simulink model "ppm_psk_shared_v3"  (R2025a)
settings: Solver=VariableStepAuto  StartTime=0.0  StopTime=5e-6  RelTol=1e-3
model workspace (MAT data in the model file):
  Sig = Simulink.Signal
  Sig.Dimensions = -1
  Sig.DimensionsMode = 'auto'
  Sig.Complexity = 'auto'
  Sig.SampleTime = -1
  Sig.SamplingMode = 'auto'
  Sig.DataType = 'auto'
  Var = 0
  fc = 4000000000
  fs = 32000000000
  fsymbol = 500000000
  ppm_spacings2_ps = [-51.8 33.2 115.3 201.3 293.8 377.9 462.9 544.9]
  ppm_spacings_ps = [698 782 869 950 1045 1127 1210 1299]
  up_fs = 1024000000000
undefined symbols (not defined in the file or in its folder): PSK
libraries: dspsigops x11, simulink_extras x7, dspstat3 x5, commsink2 x3, dspfdesign x3, commchan3 x2, commrfcorlib x1, commdigbbndpm3 x1
settings Model: ParameterArgumentNames=ppm_spacings2_ps,ppm_spacings_ps  Creator=IWMAI  LastModifiedBy=IWMAI

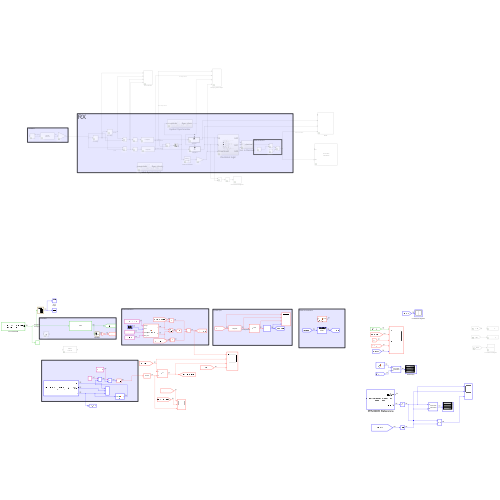
[thumbnail: Simulink's stored preview of the top-level diagram]
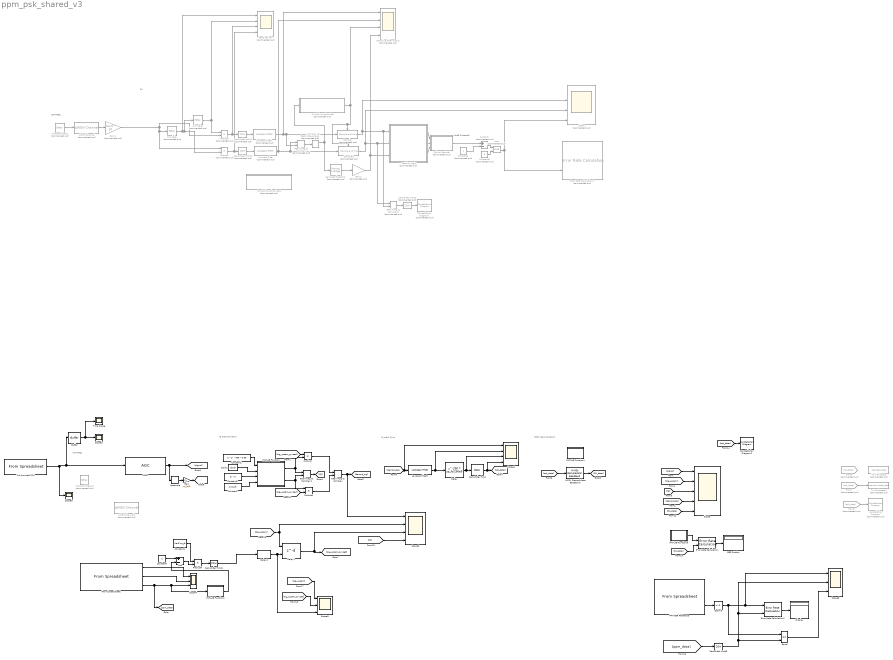
== system ppm_psk_shared_v3 ==
  note: Symbol Sync
  note: IQ Demodulation
  note: 8PSK Demodulation
  note: CHANNEL
  note: Mod8 Subtract1
  note: RX
  note: CHANNEL
  1ns trimmed PPM : FromSpreadsheet  FileName=C:\Users\IWMAI\University of Toronto\Yu Huang - Summer-2025-sharted\Yongkang\v5_250626\csv\phase_noise_ppm32.csv  SheetName=phase_noise_ppm32  SampleTime=1/fs  InterpolationWithinTimeRange=Zero order hold
  2ns delay : TransportDelay  Commented=on  DelayTime=1/fsymbol  FixedBuffer=on
  3bit to Decimal : Subsystem  Commented=on
  AGC1 : commrfcorlib/AGC  LegacyMode=off  DetectorMethod=Rectifier  LoopMethod=Linear  UpdatePeriod=100  StepSize=0.1  AdaptationStepSize=0.01  DesiredOutputPower=1  AveragingLength=100  MaximumGain=30  MaxPowerGain=60  GainOutputPort=off  InputPowerOutputPort=off  SimulateUsing=Interpreted execution
  AWGN Channel : commchan3/AWGN Channel  Commented=on  LegacyMode=off  NoiseMethod="Signal to noise ratio  (SNR)"  noiseMode="Signal to noise ratio  (SNR)"  EbNo=10  EsNo=10  SNR=16  BitsPerSymbol=1  SignalPower=1  SpecifySymbolPeriod=off  SamplesPerSymbol=1  SymbolPeriod=1  VarianceSource=Parameter  Variance=1  RandomStream=Global stream  Seed=67  SimulateUsing=Code generation
  AWGN Channel1 : commchan3/AWGN Channel  Commented=on  LegacyMode=off  NoiseMethod="Signal to noise ratio  (SNR)"  noiseMode="Signal to noise ratio  (SNR)"  EbNo=10  EsNo=10  SNR=16  BitsPerSymbol=1  SignalPower=3e-3  SpecifySymbolPeriod=off  SamplesPerSymbol=1  SymbolPeriod=1  VarianceSource=Parameter  Variance=1  RandomStream=Global stream  Seed=67  SimulateUsing=Code generation
  Add : Sum  Inputs=+-
  BER Display : Display
  Buffer : Buffer  N=32  OutputFrames=off
  Calibrate threshold : dspstat3/Moving Average  Commented=on  Method=Sliding window  ForgettingFactorPort=off  SpecifyWindowLength=on  WindowLength=10*fs/fsymbol  OverlapLength=10*fs/fsymbol - 1  AllowArbitraryInputLength=off  ForgettingFactor=0.9  SimulateUsing=Interpreted execution
  Clock1 : simulink_extras/Flip Flops/Clock  period=1/500e6
  Complex to Magnitude-Angle1 : ComplexToMagnitudeAngle  Commented=on
  Constant : Constant  Value=1/up_fs
  Constant1 : Constant  Value=2 * pi * 4e9 * 0.99
  Constant2 : Constant  Value=pi * 0
  Constant4 : Constant  Value=1e-9*up_fs
  Constant5 : Constant  Commented=on  Value=8
  Constant6 : Constant  Commented=on
  Constant7 : Constant  Value=2
  Constellation Diagram : ConstellationDiagram  Commented=on  WindowPosition=[70.000000,304.000000,385.000000,254.000000,]  ScopeFrameLocation=window  SymbolsToDisplaySource=Property  SymbolsToDisplay=2500  ReferenceConstellation=8-PSK  XLimits=[-2.067197093509777,2.1540515483355467]  YLimits=[-2.067197093509777,2.1540515483355467]  AxesLimits=[-2.067197093509777,2.1540515483355467]  EnableMeasurements=on  DefaultConfigurationName=comm.scopes.ConstellationDiagramBlockCfg
  Constellation Diagram1 : ConstellationDiagram  Commented=on  WindowPosition=[363.000000,63.000000,600.000000,600.000000,]  ScopeFrameLocation=window  SymbolsToDisplaySource=Property  SymbolsToDisplay=1000  XLimits=[-1.58,1.61]  YLimits=[-1.58,1.61]  AxesLimits=[-1.58,1.61]  EnableMeasurements=on
  Constellation Diagram2 : ConstellationDiagram  WindowPosition=[198.000000,182.000000,773.000000,552.000000,]  ScopeFrameLocation=window  SymbolsToDisplaySource=Property  SymbolsToDisplay=2500  ShowLegend=on  MaximizeAxes=on  DefaultConfigurationName=comm.scopes.ConstellationDiagramBlockCfg
  Datas : Scope  Commented=on  NumInputPorts=4
      settings: ActiveDisplayYMinimum=-0.875  ActiveDisplayYMaximum=7.875  DataLoggingVariableName=ScopeData4
  Decision logic : Subsystem  Commented=on
  Delay : Delay  DelayLength=290 * up_fs/256e9  DelayLengthUpperLimit=512  InputProcessing=Columns as channels (frame based)
  Delay1 : Delay  DelayLengthSource=Input port  DelayLength=1  DelayLengthUpperLimit=2*up_fs/1e9  InputProcessing=Columns as channels (frame based)
      settings: InputPortMap=u0,p1
  Delay2 : Delay  DelayLength=1e-9*up_fs
  Delay3 : Delay  DelayLength=0
  Display : Display
  Equal : RelationalOperator  Operator===  OutDataTypeStr=boolean  RndMeth=Simplest  InputSameDT=off
  Error Rate Calculation : commsink2/Error Rate Calculation  N=0  st_delay=0  cp_mode=Entire frame  subframe=[]  PMode=Port  WsName=ErrorVec  RsMode2=off  stop=off  numErr=100  maxBits=1e6
      settings: LibrarySourceBlock=|
      | commhdlsink/Error Rate
      | Calculation
  Error Rate Calculation1 : commsink2/Error Rate Calculation  Commented=on  N=1  st_delay=0  cp_mode=Entire frame  subframe=[]  PMode=Workspace  WsName=ErrorVec  RsMode2=off  stop=off  numErr=100  maxBits=1e6
  Error Rate Calculation2 : commsink2/Error Rate Calculation  N=0  st_delay=0  cp_mode=Entire frame  subframe=[]  PMode=Port  WsName=ErrorVec  RsMode2=off  stop=off  numErr=100  maxBits=1e6
      settings: LibrarySourceBlock=|
      | commhdlsink/Error Rate
      | Calculation
  From Spreadsheet : FromSpreadsheet  FileName=C:\Users\IWMAI\University of Toronto\Yu Huang - Summer-2025-sharted\Yongkang\v5_250626\csv\ppm_decode.csv  SheetName=ppm_decode  TreatFirstColumnAs=Data  SampleTime=1/fsymbol
  From7 : From  Commented=on  GotoTag=psk_data
  From8 : From  Commented=on  GotoTag=psk_data
  From9 : From  Commented=on  GotoTag=RX_data
  Gain : Gain  Gain=up_fs/fs
  Gain1 : Gain  Commented=on  Gain=rand * 10
  Gain2 : Gain  Commented=on  Gain=1/sqrt(2)
  Lowpass Filter : dspfdesign/Lowpass Filter  Commented=on  FilterType=FIR  DesignForMinimumOrder=on  FilterOrder=50  PassbandFrequency=0.05*fc  StopbandFrequency=0.6*fc  PassbandRipple=0.1  StopbandAttenuation=80  SampleRateMode=Specify on dialog  SampleRate=fs  SimulateUsing=Interpreted execution  roundingMode=Floor  coeffsDataTypeStr=fixdt(1,16)
  Lowpass Filter1 : dspfdesign/Lowpass Filter  Commented=on  FilterType=FIR  DesignForMinimumOrder=on  FilterOrder=50  PassbandFrequency=0.05*fc  StopbandFrequency=0.6*fc  PassbandRipple=0.1  StopbandAttenuation=80  SampleRateMode=Specify on dialog  SampleRate=fs  SimulateUsing=Interpreted execution  roundingMode=Floor  coeffsDataTypeStr=fixdt(1,16)
  Lowpass Filter3 : dspfdesign/Lowpass Filter  FilterType=FIR  DesignForMinimumOrder=on  FilterOrder=50  PassbandFrequency=0.05*fc  StopbandFrequency=0.6*fc  PassbandRipple=0.1  StopbandAttenuation=80  SampleRate=fs  SimulateUsing=Interpreted execution  roundingMode=Floor  coeffsDataTypeStr=fixdt(1,16)
  M-PSK Demodulator Baseband : commdigbbndpm3/M-PSK Demodulator Baseband  M=8  OutType=Integer  DecType=Hard decision  VarSource=Dialog  Variance=1  Dec=Gray  Mapping=[0:7]  Ph=pi/8  outDtype1=Inherit via internal rule  outDtype2=Inherit via internal rule  derotateFactorWordLen=16  derotateFactorDataTypeStr=Inherit: Same word length as input  derotateFactorLastDataTypeStr=Inherit: Same word length as input
      settings: LibrarySourceBlock=|
      | commhdldigbbndpm/M-PSK
      | Demodulator
      | Baseband
  MATLAB Function : MATLAB Function  TreatAsAtomicUnit=on  SystemSampleTime=1/up_fs
  MATLAB Function1 : MATLAB Function  TreatAsAtomicUnit=on
  MATLAB Function3 : MATLAB Function  TreatAsAtomicUnit=on  SystemSampleTime=1/500e6
  MATLAB Function4 : MATLAB Function  TreatAsAtomicUnit=on
  Mod : Math  Commented=on  Operator=mod
  PPM BER Reference : FromSpreadsheet  FileName=C:\Users\IWMAI\University of Toronto\Yu Huang - Summer-2025-sharted\Yongkang\v5_250626\csv\ground_truth_ppm.csv  SheetName=ground_truth_ppm  TreatFirstColumnAs=Data  SampleTime=1/fsymbol
  Product : Product
  Product1 : Product
  Product2 : Product  Commented=on
  Product3 : Product  Commented=on
  Product4 : Product
  Real-Imag to Complex : RealImagToComplex
  Real-Imag to Complex1 : RealImagToComplex
  Real-Imag to Complex2 : RealImagToComplex  Commented=on
  Real-Imag to Complex3 : RealImagToComplex  Commented=on
  Received raw : Scope  Commented=on  NumInputPorts=4
      settings: ActiveDisplayYMinimum=-8.64062  ActiveDisplayYMaximum=9.0483  DataLoggingVariableName=ScopeData5
  Sampler : dspsigops/Sample and Hold  Commented=on  trig=Rising edge  initCond=0  latchinput=off
  Sampler1 : dspsigops/Sample and Hold  Commented=on  trig=Rising edge  initCond=0  latchinput=off
  Sampling Filter output : Scope  Commented=on  NumInputPorts=4
      settings: ActiveDisplayYMinimum=-6.30438  ActiveDisplayYMaximum=6.9861  DataLoggingVariableName=ScopeData6
  Scope : Scope  NumInputPorts=5
      settings: ActiveDisplayYMinimum=-3.2971710288295304  ActiveDisplayYMaximum=3.6439303524490732
  Scope1 : Scope  NumInputPorts=4
      settings: ActiveDisplayYMinimum=-217.12328360095091  ActiveDisplayYMaximum=190.25679951109339  DataLoggingVariableName=ScopeData3
  Scope2 : Scope
      settings: ActiveDisplayYMinimum=-1  ActiveDisplayYMaximum=1  DataLoggingVariableName=ScopeData7
  Scope3 : Scope  NumInputPorts=4
      settings: ActiveDisplayYMinimum=-121.24929806481079  ActiveDisplayYMaximum=113.85916593857471  DataLoggingVariableName=ScopeData11
  Scope4 : Scope  NumInputPorts=3
      settings: ActiveDisplayYMinimum=-62.374999999999986  ActiveDisplayYMaximum=561.375  DataLoggingVariableName=ScopeData13
  Scope5 : Scope
      settings: ActiveDisplayYMinimum=-3.5739980150661266  ActiveDisplayYMaximum=0.60767584738395508  DataLoggingVariableName=ScopeData14
  Scope8 : Scope  NumInputPorts=3
      settings: ActiveDisplayYMinimum=-0.87499999999999978  ActiveDisplayYMaximum=7.875  DataLoggingVariableName=ScopeData17
  Scope9 : Scope  NumInputPorts=3
      settings: ActiveDisplayYMinimum=-2041.2616026203843  ActiveDisplayYMaximum=448.10816733090951  DataLoggingVariableName=ScopeData18
  Subtract : Sum  Commented=on  Inputs=+-
  Symbol Synchronizer : Subsystem  Commented=on
  Symbol Synchronizer1 : Subsystem  Commented=on
  Time Scope : Scope
      settings: TimeUnits=Metric (based on Time Span)  ActiveDisplayYMinimum=-0.20228703271248236  ActiveDisplayYMaximum=0.23303505029941141  YLabel=Amplitude  DataLoggingVariableName=ScopeData8
  To Workspace : ToWorkspace  Commented=on  VariableName=decoded_data  SaveFormat=Structure With Time  SampleTime=-1
  To Workspace1 : ToWorkspace  Commented=on  VariableName=demodulated_data  SaveFormat=Structure With Time  SampleTime=-1
  Transport Delay : TransportDelay  Commented=on  DelayTime=rand * pi/fsymbol
  Transport Delay3 : TransportDelay  Commented=on  DelayTime=rand * pi/fsymbol
  Upsample : dspsigops/Upsample  FactorSource=Dialog parameter  N=up_fs/fs  Nmax=16  phase=0  RateOptions=Allow multirate processing  ic=0  mode=Unused parameter value
      settings: LibrarySourceBlock=dsphdlsupportsigops/Upsample
  Zero-Order Hold : ZeroOrderHold  SampleTime=1/fsymbol
  Zero-Order Hold1 : ZeroOrderHold  Commented=on  SampleTime=1/fsymbol
  Zero-Order Hold2 : ZeroOrderHold  Commented=on  SampleTime=1/fs
  Zero-Order Hold3 : ZeroOrderHold  Commented=on  SampleTime=1/fs
  Zero-Order Hold4 : ZeroOrderHold  SampleTime=1/up_fs
  Zero-Order Hold5 : ZeroOrderHold  SampleTime=1/fsymbol
  pi/2 delay : TransportDelay  Commented=on  DelayTime=1/(fc)/4  FixedBuffer=on
  wires:
  From8/1 -> Constellation Diagram/1
  MATLAB Function3/1(y) -> Error Rate Calculation/1
  Error Rate Calculation/1 -> BER Display/1
  2ns delay/1 -> Product2/2, pi/2 delay/1, Received raw/1  "I p ath"
  Symbol Synchronizer/1(Sync. clock) -> Sampling Filter output/3, Sampler/Trigger, Sampler1/Trigger
  Sampler/1 -> Real-Imag to Complex3/2, Decision logic/1(Q), Datas/2
  Mod/1 -> Error Rate Calculation1/2, Datas/4  "Recovered data"
  pi/2 delay/1 -> Received raw/2, Product3/1  "Q path"
  3bit to Decimal/1(decimal) -> Subtract/1
  Decision logic/2(bit1) -> 3bit to Decimal/2(In2)
  Sampler1/1 -> Datas/3, Real-Imag to Complex3/1, Decision logic/2(I)
  Product3/1 -> Zero-Order Hold2/1, Received raw/3
  Decision logic/3(bit2) -> 3bit to Decimal/3(In3)
  Complex to Magnitude-Angle1/1 -> Symbol Synchronizer/1(magnitude), Calibrate threshold/1
  AWGN Channel/1 -> Gain1/1  "RX"
  Zero-Order Hold3/1 -> Lowpass Filter/1
  Transport Delay/1 -> AWGN Channel/1  "RX Signal"
  Subtract/1 -> Mod/1
  Real-Imag to Complex2/1 -> Complex to Magnitude-Angle1/1
  Lowpass Filter/1 -> Real-Imag to Complex2/1, Sampler1/1, Sampling Filter output/2  "no delay filtered"
  Constant5/1 -> Mod/2
  Gain2/1 -> Sampling Filter output/4, Decision logic/3(threshhold)
  Calibrate threshold/1 -> Gain2/1
  Product2/1 -> Zero-Order Hold3/1, Received raw/4
  Gain1/1 -> Product2/1, 2ns delay/1, Product3/2
  Constant6/1 -> Subtract/2
  Decision logic/1(bit0) -> 3bit to Decimal/1(In1)
  Zero-Order Hold1/1 -> Constellation Diagram1/1
  Real-Imag to Complex3/1 -> Zero-Order Hold1/1
  Zero-Order Hold2/1 -> Lowpass Filter1/1
  Lowpass Filter1/1 -> Sampling Filter output/1, Real-Imag to Complex2/2, Sampler/1  "90o delay filtered"
  [signal] -> Scope/1
  [IQ] -> Scope/3
  [demod_sig] -> Scope1/1, Lowpass Filter3/1
  Zero-Order Hold/1 -> Scope1/4, [psk_data]
  [psk_data] -> M-PSK Demodulator Baseband/1
  From7/1 -> To Workspace1/1
  M-PSK Demodulator Baseband/1 -> [RX_data]
  [RX_data] -> Error Rate Calculation/2
  Real-Imag to Complex1/1 -> [IQ]
  Constant1/1 -> MATLAB Function/1(omega)
  Clock1/1 -> MATLAB Function/2(clock)
  Constant2/1 -> MATLAB Function/3(phase_shift)
  MATLAB Function/1(I) -> Real-Imag to Complex1/1, Product/2
  MATLAB Function/2(Q) -> Product1/1, Real-Imag to Complex1/2
  [sig_upsam_synced] -> Product/1
  [sig_upsam_synced] -> Product1/2
  Product/1 -> Real-Imag to Complex/1
  Product1/1 -> Real-Imag to Complex/2
  Real-Imag to Complex/1 -> Scope3/1, [demod_sig]
  [demod_sig] -> Scope/4
  [RX_data] -> Scope/5
  1ns trimmed PPM/1 -> AGC1/1, Buffer/1, Scope5/1  "RX Signal"
  AGC1/1 -> Upsample/1, [signal]
  Buffer/1 -> Time Scope/1, Scope2/1
  Constant/1 -> MATLAB Function/4(delta_time)
  Lowpass Filter3/1 -> Scope1/2, Delay/1  "no delay filtered"
  Upsample/1 -> Gain/1
  [sig_upsam] -> Scope/2
  From Spreadsheet/1 -> Scope4/1
  From Spreadsheet/2 -> Scope4/2
  From Spreadsheet/3 -> [ppm_data], MATLAB Function1/1(index), Scope4/3
  Constant4/1 -> Product4/1
  Constant7/1 -> Add/1
  Add/1 -> Product4/2
  Delay/1 -> Scope1/3, Zero-Order Hold/1
  Product4/1 -> Zero-Order Hold4/1
  [sig_upsam] -> Delay1/1, Scope3/2
  Delay1/1 -> [sig_upsam_synced], Scope3/3
  Zero-Order Hold4/1 -> Delay2/1
  Delay2/1 -> Scope9/3, Delay1/2
  [psk_data] -> Constellation Diagram2/1
  Gain/1 -> [sig_upsam]
  [IQ] -> Scope3/4
  PPM BER Reference/2 -> Delay3/1
  Equal/1 -> Scope8/3
  Error Rate Calculation2/1 -> Display/1
  Zero-Order Hold5/1 -> Scope8/2, Error Rate Calculation2/2, Equal/2
  Delay3/1 -> Scope8/1, Error Rate Calculation2/1, Equal/1
  [ppm_data] -> Zero-Order Hold5/1
  [sig_upsam] -> Scope9/1
  [sig_upsam_synced] -> Scope9/2
  MATLAB Function1/1(y) -> Add/2

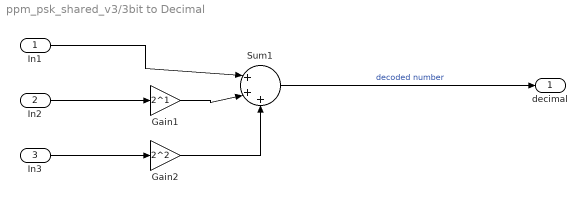
== system ppm_psk_shared_v3/3bit to Decimal ==
  In1 : Inport
  In2 : Inport  Port=2
  In3 : Inport  Port=3
  Gain1 : Gain  Gain=2^1
  Gain2 : Gain  Gain=2^2
  Sum1 : Sum  Inputs=|+++
  decimal : Outport
  wires:
  Gain2/1 -> Sum1/3
  Gain1/1 -> Sum1/2
  In3/1 -> Gain2/1
  In1/1 -> Sum1/1
  In2/1 -> Gain1/1
  Sum1/1 -> decimal/1  "decoded number"

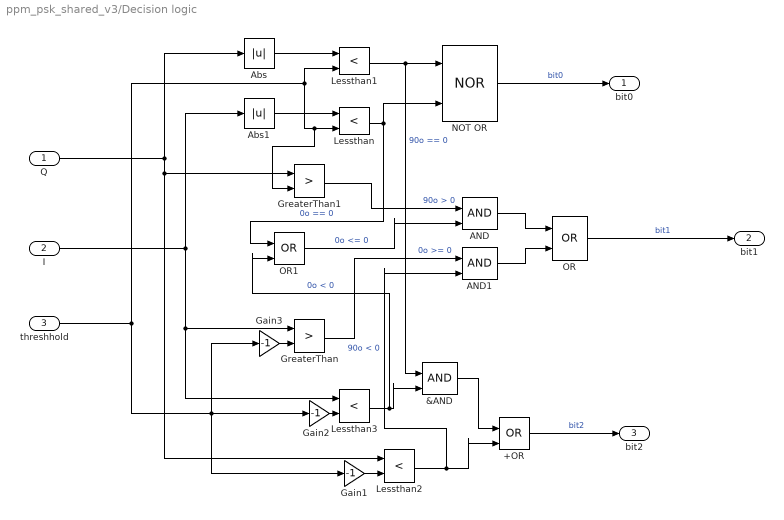
== system ppm_psk_shared_v3/Decision logic ==
  Q : Inport
  I : Inport  Port=2
  threshhold : Inport  Port=3
  &AND : Logic  IconShape=distinctive  AllPortsSameDT=off  OutDataTypeStr=boolean
  +OR : Logic  Operator=OR  IconShape=distinctive  AllPortsSameDT=off  OutDataTypeStr=boolean
  AND : Logic  IconShape=distinctive  AllPortsSameDT=off  OutDataTypeStr=boolean
  AND1 : Logic  IconShape=distinctive  AllPortsSameDT=off  OutDataTypeStr=boolean
  Abs : Abs  SaturateOnIntegerOverflow=off
  Abs1 : Abs  SaturateOnIntegerOverflow=off
  Gain1 : Gain  Gain=-1
  Gain2 : Gain  Gain=-1
  Gain3 : Gain  Gain=-1
  GreaterThan : RelationalOperator  Operator=>  OutDataTypeStr=boolean  RndMeth=Simplest  InputSameDT=off
  GreaterThan1 : RelationalOperator  Operator=>  OutDataTypeStr=boolean  RndMeth=Simplest  InputSameDT=off
  "Lessthan " : RelationalOperator  Operator=<  OutDataTypeStr=boolean  RndMeth=Simplest  InputSameDT=off
  Lessthan1 : RelationalOperator  Operator=<  OutDataTypeStr=boolean  RndMeth=Simplest  InputSameDT=off
  Lessthan2 : RelationalOperator  Operator=<  OutDataTypeStr=boolean  RndMeth=Simplest  InputSameDT=off
  Lessthan3 : RelationalOperator  Operator=<  OutDataTypeStr=boolean  RndMeth=Simplest  InputSameDT=off
  NOT OR : Logic  Operator=NOR  IconShape=distinctive  AllPortsSameDT=off  OutDataTypeStr=boolean
  OR : Logic  Operator=OR  IconShape=distinctive  AllPortsSameDT=off  OutDataTypeStr=boolean
  OR1 : Logic  Operator=OR  IconShape=distinctive  AllPortsSameDT=off  OutDataTypeStr=boolean
  bit0 : Outport
  bit1 : Outport  Port=2
  bit2 : Outport  Port=3
  wires:
  NOT OR/1 -> bit0/1  "bit0"
  Lessthan2/1 -> AND1/2, +OR/2  "90o < 0"
  "Lessthan "/1 -> OR1/1, NOT OR/2  "0o == 0"
  Abs1/1 -> "Lessthan "/1
  GreaterThan/1 -> AND1/1  "0o >= 0"
  I/1 -> Abs1/1, GreaterThan/1, Lessthan3/1
  Gain1/1 -> Lessthan2/2
  OR1/1 -> AND/2  "0o <= 0"
  GreaterThan1/1 -> AND/1  "90o > 0"
  AND/1 -> OR/1
  Q/1 -> Abs/1, Lessthan2/1, GreaterThan1/1
  Gain3/1 -> GreaterThan/2
  Lessthan3/1 -> OR1/2, &AND/2  "0o < 0"
  Abs/1 -> Lessthan1/1
  threshhold/1 -> Gain1/1, Gain2/1, Gain3/1, GreaterThan1/2, "Lessthan "/2, Lessthan1/2
  Lessthan1/1 -> NOT OR/1, &AND/1  "90o == 0"
  AND1/1 -> OR/2
  &AND/1 -> +OR/1
  Gain2/1 -> Lessthan3/2
  +OR/1 -> bit2/1  "bit2"
  OR/1 -> bit1/1  "bit1"

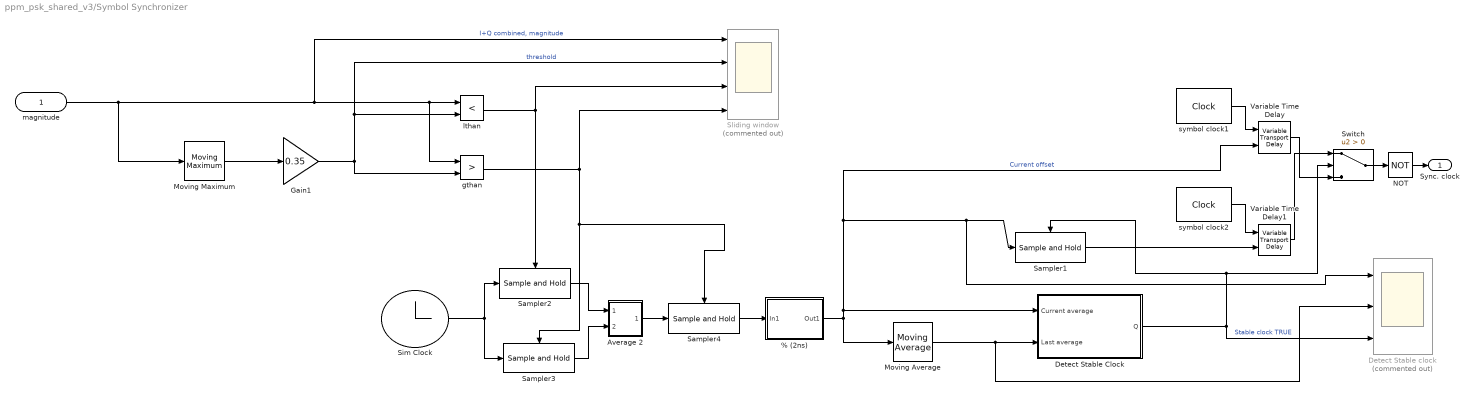
== system ppm_psk_shared_v3/Symbol Synchronizer ==
  magnitude : Inport
  % (2ns) : Subsystem
  Average 2 : Subsystem
  Detect Stable Clock : Subsystem
  Detect Stable clock : Scope  Commented=on  NumInputPorts=3
      settings: ActiveDisplayYMinimum=-1E-10  ActiveDisplayYMaximum=1.2E-9
  Gain1 : Gain  Gain=0.35
  Moving Average : dspstat3/Moving Average  Method=Sliding window  ForgettingFactorPort=off  SpecifyWindowLength=on  WindowLength=4*fs/fsymbol  OverlapLength=4*fs/fsymbol-1  AllowArbitraryInputLength=off  ForgettingFactor=0.9  SimulateUsing=Interpreted execution
  Moving Maximum : dspstat3/Moving Maximum  SpecifyWindowLength=on  WindowLength=2*fs/fsymbol  SimulateUsing=Interpreted execution
  NOT : Logic  Operator=NOT  IconShape=distinctive  AllPortsSameDT=off  OutDataTypeStr=boolean
  Sampler{1..4} (4 alike) : dspsigops/Sample and Hold  trig=Rising edge  initCond=0  latchinput=off
  Sim Clock : Clock
  Sliding window : Scope  Commented=on  NumInputPorts=4
      settings: ActiveDisplayYMinimum=-1.49431  ActiveDisplayYMaximum=13.44875  DataLoggingVariableName=ScopeData2
  Switch : Switch  Criteria=u2 > Threshold  SaturateOnIntegerOverflow=off  InputSameDT=off
  Variable Time Delay : VariableTransportDelay  MaximumDelay=10
  Variable Time Delay1 : VariableTransportDelay  MaximumDelay=10
  gthan : RelationalOperator  Operator=>  OutDataTypeStr=boolean  RndMeth=Simplest  InputSameDT=off
  lthan : RelationalOperator  Operator=<  OutDataTypeStr=boolean  RndMeth=Simplest  InputSameDT=off
  symbol clock1 : simulink_extras/Flip Flops/Clock  period=1/fsymbol
  symbol clock2 : simulink_extras/Flip Flops/Clock  period=1/fsymbol
  Sync. clock : Outport
  wires:
  Sim Clock/1 -> Sampler2/1, Sampler3/1
  Sampler3/1 -> Average 2/2(In2)
  Gain1/1 -> gthan/2, Sliding window/2, lthan/2  "threshold"
  Sampler2/1 -> Average 2/1(In1)
  symbol clock1/1 -> Variable Time Delay/1
  Sampler4/1 -> % (2ns)/1(In1)
  lthan/1 -> Sampler2/Trigger, Sliding window/3
  Average 2/1(Out1) -> Sampler4/1
  magnitude/1 -> Moving Maximum/1, Sliding window/1, gthan/1, lthan/1  "I+Q combined, magnitude"
  gthan/1 -> Sampler4/Trigger, Sampler3/Trigger, Sliding window/4
  symbol clock2/1 -> Variable Time Delay1/1
  Sampler1/1 -> Variable Time Delay1/2
  Switch/1 -> NOT/1
  Variable Time Delay/1 -> Switch/3
  Variable Time Delay1/1 -> Switch/1
  NOT/1 -> Sync. clock/1
  Detect Stable Clock/1(Q) -> Detect Stable clock/3, Sampler1/Trigger, Switch/2  "Stable clock TRUE"
  % (2ns)/1(Out1) -> Variable Time Delay/2, Detect Stable clock/1, Sampler1/1, Detect Stable Clock/1(Current average), Moving Average/1  "Current offset"
  Moving Maximum/1 -> Gain1/1
  Moving Average/1 -> Detect Stable clock/2, Detect Stable Clock/2(Last average)

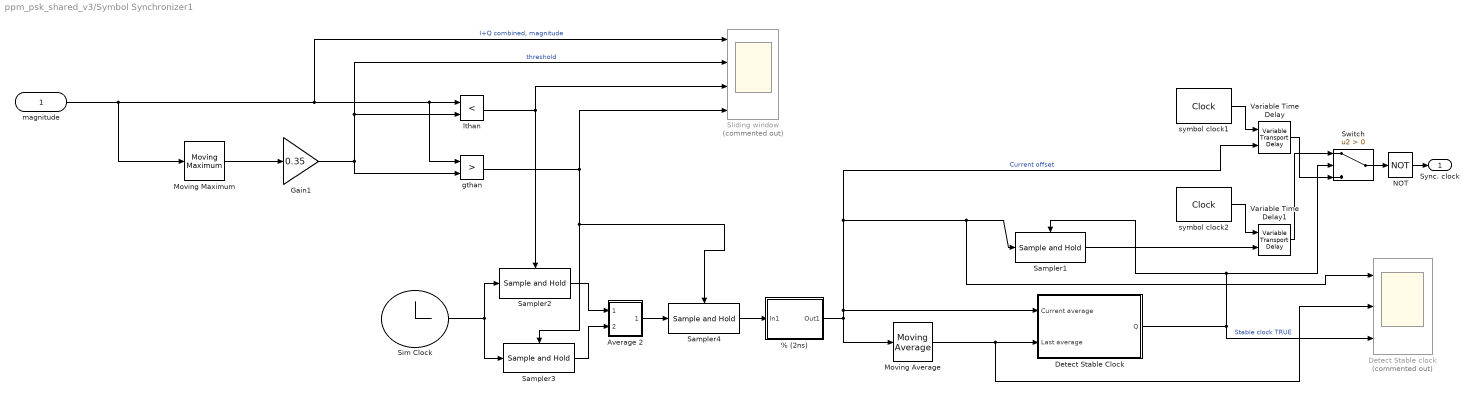
== system ppm_psk_shared_v3/Symbol Synchronizer1 ==
  magnitude : Inport
  % (2ns) : Subsystem
  Average 2 : Subsystem
  Detect Stable Clock : Subsystem
  Detect Stable clock : Scope  Commented=on  NumInputPorts=3
      settings: ActiveDisplayYMinimum=-1E-10  ActiveDisplayYMaximum=1.2E-9
  Gain1 : Gain  Gain=0.35
  Moving Average : dspstat3/Moving Average  Method=Sliding window  ForgettingFactorPort=off  SpecifyWindowLength=on  WindowLength=4*fs/fsymbol  OverlapLength=4*fs/fsymbol-1  AllowArbitraryInputLength=off  ForgettingFactor=0.9  SimulateUsing=Interpreted execution
  Moving Maximum : dspstat3/Moving Maximum  SpecifyWindowLength=on  WindowLength=2*fs/fsymbol  SimulateUsing=Interpreted execution
  NOT : Logic  Operator=NOT  IconShape=distinctive  AllPortsSameDT=off  OutDataTypeStr=boolean
  Sampler{1..4} (4 alike) : dspsigops/Sample and Hold  trig=Rising edge  initCond=0  latchinput=off
  Sim Clock : Clock
  Sliding window : Scope  Commented=on  NumInputPorts=4
      settings: ActiveDisplayYMinimum=-1.49431  ActiveDisplayYMaximum=13.44875  DataLoggingVariableName=ScopeData2
  Switch : Switch  Criteria=u2 > Threshold  SaturateOnIntegerOverflow=off  InputSameDT=off
  Variable Time Delay : VariableTransportDelay  MaximumDelay=10
  Variable Time Delay1 : VariableTransportDelay  MaximumDelay=10
  gthan : RelationalOperator  Operator=>  OutDataTypeStr=boolean  RndMeth=Simplest  InputSameDT=off
  lthan : RelationalOperator  Operator=<  OutDataTypeStr=boolean  RndMeth=Simplest  InputSameDT=off
  symbol clock1 : simulink_extras/Flip Flops/Clock  period=1/fsymbol
  symbol clock2 : simulink_extras/Flip Flops/Clock  period=1/fsymbol
  Sync. clock : Outport
  wires:
  Sim Clock/1 -> Sampler2/1, Sampler3/1
  Sampler3/1 -> Average 2/2(In2)
  Gain1/1 -> gthan/2, Sliding window/2, lthan/2  "threshold"
  Sampler2/1 -> Average 2/1(In1)
  symbol clock1/1 -> Variable Time Delay/1
  Sampler4/1 -> % (2ns)/1(In1)
  lthan/1 -> Sampler2/Trigger, Sliding window/3
  Average 2/1(Out1) -> Sampler4/1
  magnitude/1 -> Moving Maximum/1, Sliding window/1, gthan/1, lthan/1  "I+Q combined, magnitude"
  gthan/1 -> Sampler4/Trigger, Sampler3/Trigger, Sliding window/4
  symbol clock2/1 -> Variable Time Delay1/1
  Sampler1/1 -> Variable Time Delay1/2
  Switch/1 -> NOT/1
  Variable Time Delay/1 -> Switch/3
  Variable Time Delay1/1 -> Switch/1
  NOT/1 -> Sync. clock/1
  Detect Stable Clock/1(Q) -> Detect Stable clock/3, Sampler1/Trigger, Switch/2  "Stable clock TRUE"
  % (2ns)/1(Out1) -> Variable Time Delay/2, Detect Stable clock/1, Sampler1/1, Detect Stable Clock/1(Current average), Moving Average/1  "Current offset"
  Moving Maximum/1 -> Gain1/1
  Moving Average/1 -> Detect Stable clock/2, Detect Stable Clock/2(Last average)

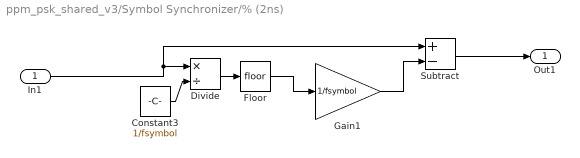
== system ppm_psk_shared_v3/Symbol Synchronizer/% (2ns) ==
  In1 : Inport
  Constant3 : Constant  Value=1/fsymbol
  Divide : Product  Inputs=*/
  Floor : Rounding
  Gain1 : Gain  Gain=1/fsymbol
  Subtract : Sum  Inputs=+-
  Out1 : Outport
  wires:
  Subtract/1 -> Out1/1
  Divide/1 -> Floor/1
  In1/1 -> Subtract/1, Divide/1
  Gain1/1 -> Subtract/2
  Floor/1 -> Gain1/1
  Constant3/1 -> Divide/2

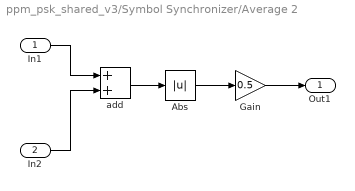
== system ppm_psk_shared_v3/Symbol Synchronizer/Average 2 ==
  In1 : Inport
  In2 : Inport  Port=2
  Abs : Abs  SaturateOnIntegerOverflow=off
  Gain : Gain  Gain=0.5
  add : Sum
  Out1 : Outport
  wires:
  Gain/1 -> Out1/1
  In1/1 -> add/1
  In2/1 -> add/2
  add/1 -> Abs/1
  Abs/1 -> Gain/1

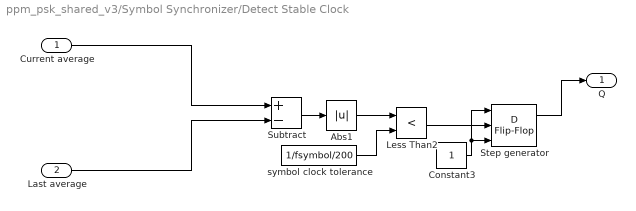
== system ppm_psk_shared_v3/Symbol Synchronizer/Detect Stable Clock ==
  Current average : Inport
  Last average : Inport  Port=2
  Abs1 : Abs  SaturateOnIntegerOverflow=off
  Constant3 : Constant  OutDataTypeStr=boolean
  Less Than2 : RelationalOperator  Operator=<  OutDataTypeStr=boolean  RndMeth=Simplest  InputSameDT=off
  Step generator : simulink_extras/Flip Flops/D Flip-Flop
  Subtract : Sum  Inputs=+-
  symbol clock tolerance : Constant  Value=1/fsymbol/200
  Q : Outport
  wires:
  symbol clock tolerance/1 -> Less Than2/2
  Subtract/1 -> Abs1/1
  Constant3/1 -> Step generator/1, Step generator/3
  Last average/1 -> Subtract/2
  Abs1/1 -> Less Than2/1
  Less Than2/1 -> Step generator/2
  Step generator/1 -> Q/1
  Current average/1 -> Subtract/1

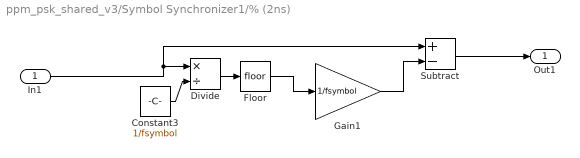
== system ppm_psk_shared_v3/Symbol Synchronizer1/% (2ns) ==
  In1 : Inport
  Constant3 : Constant  Value=1/fsymbol
  Divide : Product  Inputs=*/
  Floor : Rounding
  Gain1 : Gain  Gain=1/fsymbol
  Subtract : Sum  Inputs=+-
  Out1 : Outport
  wires:
  Subtract/1 -> Out1/1
  Divide/1 -> Floor/1
  In1/1 -> Subtract/1, Divide/1
  Gain1/1 -> Subtract/2
  Floor/1 -> Gain1/1
  Constant3/1 -> Divide/2

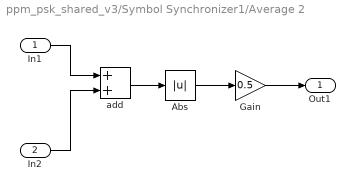
== system ppm_psk_shared_v3/Symbol Synchronizer1/Average 2 ==
  In1 : Inport
  In2 : Inport  Port=2
  Abs : Abs  SaturateOnIntegerOverflow=off
  Gain : Gain  Gain=0.5
  add : Sum
  Out1 : Outport
  wires:
  Gain/1 -> Out1/1
  In1/1 -> add/1
  In2/1 -> add/2
  add/1 -> Abs/1
  Abs/1 -> Gain/1

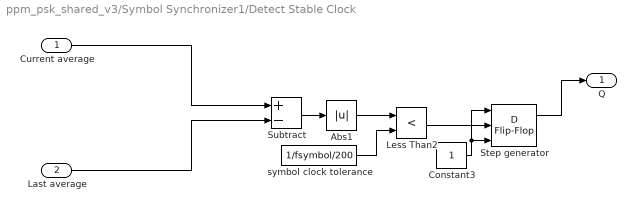
== system ppm_psk_shared_v3/Symbol Synchronizer1/Detect Stable Clock ==
  Current average : Inport
  Last average : Inport  Port=2
  Abs1 : Abs  SaturateOnIntegerOverflow=off
  Constant3 : Constant  OutDataTypeStr=boolean
  Less Than2 : RelationalOperator  Operator=<  OutDataTypeStr=boolean  RndMeth=Simplest  InputSameDT=off
  Step generator : simulink_extras/Flip Flops/D Flip-Flop
  Subtract : Sum  Inputs=+-
  symbol clock tolerance : Constant  Value=1/fsymbol/200
  Q : Outport
  wires:
  symbol clock tolerance/1 -> Less Than2/2
  Subtract/1 -> Abs1/1
  Constant3/1 -> Step generator/1, Step generator/3
  Last average/1 -> Subtract/2
  Abs1/1 -> Less Than2/1
  Less Than2/1 -> Step generator/2
  Step generator/1 -> Q/1
  Current average/1 -> Subtract/1

== matlab function ppm_psk_shared_v3/MATLAB Function1 ==
  data: index input; y output
function y = mapp(index)

map = [0.6943 0.7793 0.8663 0.9512 1.0423 1.1270 1.2079 1.2933];
map2 = [0.6922 0.7774 0.8653 0.9521 1.0420 1.1250 1.2061 1.2891];
map3 = [0.6758 0.7578 0.8474 0.9297 1.0129 1.1010 1.1836 1.2695];
map4 = [0.6769 0.7575 0.8466 0.9310 1.0135 1.1012 1.1848 1.2694];
map5 = [0.67187500 0.75683594 0.84277344 0.92773438 1.01269531 1.09808077 1.18359375 1.26793381];

y = map5(index + 1);

== matlab function ppm_psk_shared_v3/MATLAB Function ==
  data: omega input; clock input; I output; phase_shift input; Q output; delta_time input
function [I, Q]= custom_sine(omega, clock, phase_shift, delta_time)

% around 4GHz sine wave, restart 1/500e6 sec
% currently assume the sample rate is 16S/s

persistent count;
persistent last_clock; % for detecting the falling edge, because we want to reset the wave on the falling edge

if isempty(count)
    count = 0;
    last_clock = 1;
end

if clock == 0 && last_clock == 1 % means we are on a falling edge
    count = 0;
end

phase = count * omega * delta_time + phase_shift;

I = cos(phase);
Q = -sin(phase);

count = count + 1;
last_clock = clock;

== matlab function ppm_psk_shared_v3/MATLAB Function3 ==
  data: y output
function y = TX_data

persistent index;
persistent ans_buffer;

buffer_len = 127;

if isempty(index)
    index = 1;
    ans_buffer = [7 4 2 2 2 2 2 6 5 3 3 3 3 7 2 7 5 5 5 1 0 2 1 7 7 3 6 7 0 5 3 7 6 4 4 0 7 1 4 1 7 3 6 7 4 6 5 7 6 4 0 3 4 5 6 3 5 4 2 2 2 6 1 2 7 5 5 1 0 6 2 1 7 3 6 3 5 0 5 7 6 0 3 0 2 5 6 7 4 6 1 6 4 4 0 3 0 2 1 7 3 2 4 7 0 5 7 2 3 0 6 2 5 2 0 4 3 5 4 6 5 7 2 3 4 5 6];
end

y = ans_buffer(mod(index, buffer_len) + 1);
index = index + 1;

== matlab function ppm_psk_shared_v3/MATLAB Function4 ==
  data: rx input; symIdx output
function symIdx = my_8psk_decoder(rx)
% rx: complex input symbol
% symIdx: integer index [0~7]

% 固定参考点（从 Python 得到）
persistent centers
if isempty(centers)
    centers = [
-0.794546 + -0.298444i;
-0.425530 + -0.703649i;
0.731182 + -0.125290i;
0.232761 + -0.730665i;
-0.220880 + 0.731179i;
-0.772253 + 0.362395i;
0.270349 + 0.746917i;
0.682762 + 0.402678i;
    ]; % 改成你实际的
end

% 最小距离判决
dist = abs(rx - centers);
[~, symIdx] = min(dist);

symIdx = symIdx - 1; % MATLAB index从1开始，转成0~7
